simulink model "math_vect_2_test"  (Simulink 7.2)
settings: Solver=VariableStepDiscrete  StartTime=0.0  StopTime=10.0  RelTol=1e-3
settings Model: Creator=arnaud  LastModifiedBy=arnaud
settings DataIOCC: SaveFormat=Structure

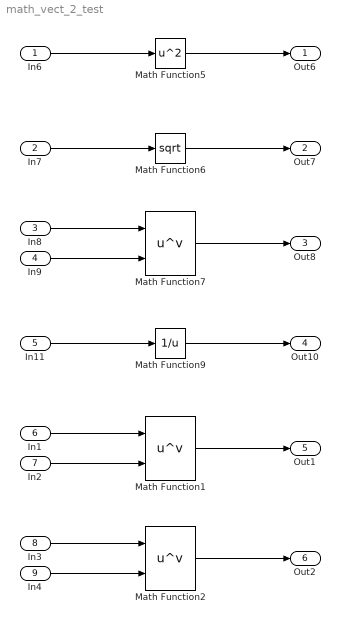
== system math_vect_2_test ==
  In6 : Inport  PortDimensions=3  OutDataType=sfix(16)  OutScaling=2^0
  In7 : Inport  Port=2  PortDimensions=3  OutDataType=sfix(16)  OutScaling=2^0
  In8 : Inport  Port=3  PortDimensions=3  OutDataType=sfix(16)  OutScaling=2^0
  In9 : Inport  Port=4  PortDimensions=3  OutDataType=sfix(16)  OutScaling=2^0
  In11 : Inport  Port=5  PortDimensions=3  OutDataType=sfix(16)  OutScaling=2^0
  In1 : Inport  Port=6  PortDimensions=3  OutDataType=sfix(16)  OutScaling=2^0
  In2 : Inport  Port=7  PortDimensions=1  OutDataType=sfix(16)  OutScaling=2^0
  In3 : Inport  Port=8  PortDimensions=1  OutDataType=sfix(16)  OutScaling=2^0
  In4 : Inport  Port=9  PortDimensions=3  OutDataType=sfix(16)  OutScaling=2^0
  Math Function1 : Math  Operator=pow  OutDataType=sfix(16)  OutScaling=2^0  SaturateOnIntegerOverflow=on
  Math Function2 : Math  Operator=pow  OutDataType=sfix(16)  OutScaling=2^0  SaturateOnIntegerOverflow=on
  Math Function5 : Math  Operator=square  OutDataType=sfix(16)  OutScaling=2^0  SaturateOnIntegerOverflow=on
  Math Function6 : Math  Operator=sqrt  OutDataType=sfix(16)  OutScaling=2^0  SaturateOnIntegerOverflow=on
  Math Function7 : Math  Operator=pow  OutDataType=sfix(16)  OutScaling=2^0  SaturateOnIntegerOverflow=on
  Math Function9 : Math  Operator=reciprocal  OutDataType=sfix(16)  OutScaling=2^0  SaturateOnIntegerOverflow=on
  Out6 : Outport  OutDataType=sfix(16)  OutScaling=2^0
  Out7 : Outport  Port=2  OutDataType=sfix(16)  OutScaling=2^0
  Out8 : Outport  Port=3  OutDataType=sfix(16)  OutScaling=2^0
  Out10 : Outport  Port=4  OutDataType=sfix(16)  OutScaling=2^0
  Out1 : Outport  Port=5  OutDataType=sfix(16)  OutScaling=2^0
  Out2 : Outport  Port=6  OutDataType=sfix(16)  OutScaling=2^0
  wires:
  In6/1 -> Math Function5/1
  Math Function5/1 -> Out6/1
  In7/1 -> Math Function6/1
  Math Function6/1 -> Out7/1
  In8/1 -> Math Function7/1
  In9/1 -> Math Function7/2
  Math Function7/1 -> Out8/1
  In11/1 -> Math Function9/1
  Math Function9/1 -> Out10/1
  In1/1 -> Math Function1/1
  In2/1 -> Math Function1/2
  Math Function1/1 -> Out1/1
  In3/1 -> Math Function2/1
  In4/1 -> Math Function2/2
  Math Function2/1 -> Out2/1
